simulink model "uart_xy_wiggler"  (R2018a)
settings: Solver=FixedStepDiscrete  StartTime=0.0  StopTime=inf  RelTol=1e-3
PreLoadFcn:
  | waijung.modelPreload; % Required for working with Waijung Blockset. Do not remove.
undefined symbols (not defined in the file or in its folder): HSEOSC, Link, LQFP144, ST, STM32F446ZE
libraries: simulink x10, commsynccomp2 x7, stm32f4_io_lib x3, dspstat3 x2, stm32f4_device_config_lib x1, dspbuff3 x1
(part 5 of 9)

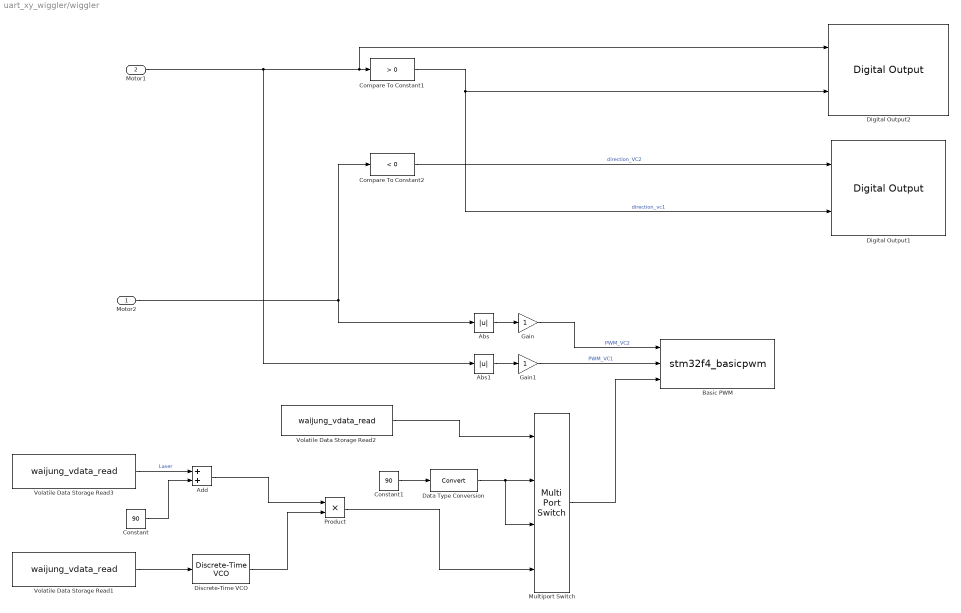
== system uart_xy_wiggler/wiggler ==
  Motor2 : Inport
  Motor1 : Inport  Port=2
  Abs : Abs
  Abs1 : Abs
  Add : Sum
  Basic PWM : S-Function  FunctionName=stm32f4_basicpwm  Parameters=timer,pwmperiod,ch1pin,ch2pin,ch3pin,ch4pin,sampletime,sampletimestr,blockid,apb,portstr,pinstr,pinmat,timarr,timprescale,chmat,polaritystr  SFunctionDeploymentMode=off  EnableBusSupport=off  mask(stm32f4_basicpwm){timer=3, pwmperiod=5.0000e-05, polarity=Active High, polaritystr=TIM_OCPolarity_High, ch1pin=Not available - Do not use, ch2pin=C7, ch3pin=C8, ch4pin=C9, sampletime=0.001, sampletimestr=-1, blockid=wigglerBasicPWM, portpinstr=,C7,C8,C9, enablecustomportlabel=off, cinputportlabel=In1, In2, In3, In4, coutputportlabel=0, apb=1, portstr=["C"], pinstr=["GPIO_Pin_7 | GPIO_Pin_8 | GPIO_Pin_9"], pinmat=[3 7 8 9], timarr=4499, timprescale=0, chmat=[2  3  4]}
      mask prompts: pwmperiod "PWM Period (seconds)"; ch1pin "Channel 1"; ch2pin "Channel 2"; ch3pin "Channel 3"; ch4pin "Channel 4"; sampletime "Sample time (sec)"; sampletimestr "Compiled sample time (sec) in string"; portpinstr "Port pin string"; enablecustomportlabel "Enable custom port labels"; cinputportlabel "Custom input port labels (Ex. In1, In2, In3)"; coutputportlabel "Custom output port labels (Ex. Out1, Out2, Out3)"; portstr "Port string"; pinstr "Pin string"; pinmat "Pin matrix"; timarr "Timer ARR"; timprescale "Timer PRESCALE"; chmat "Channel order"
      mask help:
      | This block implements basic Edge-aligned Pulse Width Modulation (PWM) generation.
      | All timers are 16-bit. The PWM period is fixed (per timer).
      mask init:
      | stm32f4_basicpwm_callback('init');
      mask Help: web(fullfile(waijungdocroot,'stm32f4_basicpwm.htm'),'-browser')
      mask TypeOptions timer: 1 | 2 | 3 | 4 | 5 | 8 | 9 | 10 | 11 | 12 | 13 | 14
      mask Callback timer: stm32f4_basicpwm_callback('timer');
      mask Callback pwmperiod: stm32f4_basicpwm_callback('pwmperiod');
      mask TypeOptions polarity: Active High | Active Low
      mask Callback polarity: stm32f4_basicpwm_callback('polarity');
      mask TypeOptions ch1pin: Not available - Do not use | A6 | B4 | C6
      mask Callback ch1pin: stm32f4_basicpwm_callback('ch1pin');
      mask TypeOptions ch2pin: Not available - Do not use | A7 | B5 | C7
      mask Callback ch2pin: stm32f4_basicpwm_callback('ch2pin');
      mask TypeOptions ch3pin: Not available - Do not use | B0 | C8
      mask Callback ch3pin: stm32f4_basicpwm_callback('ch3pin');
      mask TypeOptions ch4pin: Not available - Do not use | B1 | C9
      mask Callback ch4pin: stm32f4_basicpwm_callback('ch4pin');
      mask Callback sampletime: stm32f4_basicpwm_callback('sampletime');
      mask Callback sampletimestr: stm32f4_basicpwm_callback('sampletimestr');
      mask Callback blockid: stm32f4_basicpwm_callback('blockid');
      mask Callback enablecustomportlabel: stm32f4_basicpwm_callback('enablecustomportlabel');
      mask Display: text(0.95, 0.5, 'Timer: 3\nPolarity: Active High\nPeriod (sec) 5.0000e-05 \nTs (sec): -1','ver','middle','hor','right');port_label('input', 1,'CH2 (C7)');port_label('input', 2,'CH3 (C8)');port_label('input', 3,'CH4 (C9)')
  Compare To Constant1 : simulink/Logic and Bit Operations/Compare To Constant  relop=>  const=0  OutDataTypeStr=boolean
  Compare To Constant2 : simulink/Logic and Bit Operations/Compare To Constant  relop=<  const=0  OutDataTypeStr=boolean
  Constant : Constant  Value=90
  Constant1 : Constant  Value=90  SampleTime=0.01
  Data Type Conversion : DataTypeConversion
  Digital Output1 : stm32f4_io_lib/Digital Output  use_bitband=on  port=F  speed=100  porttype=Push Pull  porttypestr=PP  use_pin0=off  use_pin1=off  use_pin2=off  use_pin3=off  use_pin4=off  use_pin5=off  use_pin6=off  use_pin7=off  use_pin8=off  use_pin9=off  use_pin10=off  use_pin11=off  use_pin12=off  use_pin13=on  use_pin14=on  use_pin15=off  pinstr=GPIO_Pin_13 | GPIO_Pin_14  usedpinarray="[0  0  0  0  0  0  0  0  0  0  0  0  0  1  1  0]"  bitbandingstr=|  sampletime=-1  sampletimestr=-1  blockid=wigglerDigitalOutput1  enablecustomportlabel=off  globalinit=off  cinputportlabel=In1, In2  coutputportlabel=0
      | #define wigglerDigitalOutput1_F13 Peripheral_BB(GPIOF->ODR, 13)  /* Output pin */
      | #define wigglerDigitalOutput1_F14 Peripheral_BB(GPIOF->ODR, 14)  /* Output pin */
      settings: SourceProductName=Waijung Blockset
  Digital Output2 : stm32f4_io_lib/Digital Output  use_bitband=on  port=D  speed=100  porttype=Push Pull  porttypestr=PP  use_pin0=on  use_pin1=off  use_pin2=off  use_pin3=off  use_pin4=off  use_pin5=off  use_pin6=off  use_pin7=on  use_pin8=off  use_pin9=off  use_pin10=off  use_pin11=off  use_pin12=off  use_pin13=off  use_pin14=off  use_pin15=off  pinstr=GPIO_Pin_0 | GPIO_Pin_7  usedpinarray="[1  0  0  0  0  0  0  1  0  0  0  0  0  0  0  0]"  bitbandingstr=|  sampletime=-1  sampletimestr=-1  blockid=wigglerDigitalOutput2  enablecustomportlabel=off  globalinit=off  cinputportlabel=In1, In2  coutputportlabel=0
      | #define wigglerDigitalOutput2_D0 Peripheral_BB(GPIOD->ODR, 0)  /* Output pin */
      | #define wigglerDigitalOutput2_D7 Peripheral_BB(GPIOD->ODR, 7)  /* Output pin */
      settings: SourceProductName=Waijung Blockset
  Discrete-Time VCO : commsynccomp2/Discrete-Time VCO  Ac=1  Fc=0  Kc=1  Ph=0  ts=0.01
      settings: SourceProductName=Communications System Toolbox  SourceProductBaseCode=CM
  Gain : Gain
  Gain1 : Gain
  Multiport Switch : MultiPortSwitch  DataPortOrder=Zero-based contiguous  zeroidx=on
  Product : Product
  Volatile Data Storage Read1 : S-Function  FunctionName=waijung_vdata_read  Parameters=storagename,varname,sampletime,sampletimestr,blockid,storagetype,storagetypestr  SFunctionDeploymentMode=off  EnableBusSupport=off  mask(waijung_vdata_read){storagename=LissaFreq, varname=LissajousDataVolatileDataStorage8_LissaFreq, sampletime=.01, sampletimestr=-1, blockid=wigglerVolatileDataStorageRead1, storagetype=double, storagetypestr=double}
      mask prompts: storagename "Storage Name"; varname "Variable name"; sampletime "Sample time (sec)"; sampletimestr "Compiled sample time (sec) in string"; storagetype "Data type"; storagetypestr "Data type string"
      mask help: This block implements read data from a buffer.
      mask init:
      | waijung_vdata_read_callback('init');
      mask Help: web(fullfile(waijungdocroot,'Volatile_Data_Storage_Read.htm'))
      mask TypeOptions storagename: ab3 | ab1 | ab2 | ab4 | ab5 | ab6 | ab7 | ab8 | ab9 | ab10 | Ays | Ayc | Axs | A_Laser | LissaFreq | Axc | Laser | vcx | flag | CircleFlag | CircleFrequency | vcy | CircleR
      mask Callback storagename: waijung_vdata_read_callback('storagename');
      mask Callback varname: waijung_vdata_read_callback('varname');
      mask Callback sampletime: waijung_vdata_read_callback('sampletime');
      mask Callback sampletimestr: waijung_vdata_read_callback('sampletimestr');
      mask Callback blockid: waijung_vdata_read_callback('blockid');
      mask Callback storagetype: waijung_vdata_read_callback('storagetype');
      mask Display: text(0.05, 0.5, 'Buffer: LissaFreq','ver','middle','hor','left');port_label('output',1,'D1(double)')
  Volatile Data Storage Read2 : S-Function  FunctionName=waijung_vdata_read  Parameters=storagename,varname,sampletime,sampletimestr,blockid,storagetype,storagetypestr  SFunctionDeploymentMode=off  EnableBusSupport=off  mask(waijung_vdata_read){storagename=CircleFlag, varname=VolatileDataStorage4_CircleFlag, sampletime=.01, sampletimestr=-1, blockid=VolatileDataStorageRead2, storagetype=double, storagetypestr=double}
      mask prompts: storagename "Storage Name"; varname "Variable name"; sampletime "Sample time (sec)"; sampletimestr "Compiled sample time (sec) in string"; storagetype "Data type"; storagetypestr "Data type string"
      mask help: This block implements read data from a buffer.
      mask init:
      | waijung_vdata_read_callback('init');
      mask Help: web(fullfile(waijungdocroot,'Volatile_Data_Storage_Read.htm'))
      mask TypeOptions storagename: ab3 | ab1 | ab2 | ab4 | ab5 | ab6 | ab7 | ab8 | ab9 | ab10 | Ays | Ayc | Axs | A_Laser | LissaFreq | Axc | Laser | vcx | flag | CircleFlag | CircleFrequency | vcy | CircleR
      mask Callback storagename: waijung_vdata_read_callback('storagename');
      mask Callback varname: waijung_vdata_read_callback('varname');
      mask Callback sampletime: waijung_vdata_read_callback('sampletime');
      mask Callback sampletimestr: waijung_vdata_read_callback('sampletimestr');
      mask Callback blockid: waijung_vdata_read_callback('blockid');
      mask Callback storagetype: waijung_vdata_read_callback('storagetype');
      mask Display: text(0.05, 0.5, 'Buffer: CircleFlag','ver','middle','hor','left');port_label('output',1,'D1(double)')
  Volatile Data Storage Read3 : S-Function  FunctionName=waijung_vdata_read  Parameters=storagename,varname,sampletime,sampletimestr,blockid,storagetype,storagetypestr  SFunctionDeploymentMode=off  EnableBusSupport=off  mask(waijung_vdata_read){storagename=A_Laser, varname=LissajousDataVolatileDataStorage7_A_Laser, sampletime=.01, sampletimestr=-1, blockid=wigglerVolatileDataStorageRead3, storagetype=double, storagetypestr=double}
      mask prompts: storagename "Storage Name"; varname "Variable name"; sampletime "Sample time (sec)"; sampletimestr "Compiled sample time (sec) in string"; storagetype "Data type"; storagetypestr "Data type string"
      mask help: This block implements read data from a buffer.
      mask init:
      | waijung_vdata_read_callback('init');
      mask Help: web(fullfile(waijungdocroot,'Volatile_Data_Storage_Read.htm'))
      mask TypeOptions storagename: ab3 | ab1 | ab2 | ab4 | ab5 | ab6 | ab7 | ab8 | ab9 | ab10 | Ays | Ayc | Axs | A_Laser | LissaFreq | Axc | Laser | vcx | flag | CircleFlag | CircleFrequency | vcy | CircleR
      mask Callback storagename: waijung_vdata_read_callback('storagename');
      mask Callback varname: waijung_vdata_read_callback('varname');
      mask Callback sampletime: waijung_vdata_read_callback('sampletime');
      mask Callback sampletimestr: waijung_vdata_read_callback('sampletimestr');
      mask Callback blockid: waijung_vdata_read_callback('blockid');
      mask Callback storagetype: waijung_vdata_read_callback('storagetype');
      mask Display: text(0.05, 0.5, 'Buffer: A_Laser','ver','middle','hor','left');port_label('output',1,'D1(double)')
  wires:
  Gain1/1 -> Basic PWM/2  "PWM_VC1"
  Gain/1 -> Basic PWM/1  "PWM_VC2"
  Compare To Constant1/1 -> Digital Output1/2, Digital Output2/2  "direction_vc1"
  Compare To Constant2/1 -> Digital Output1/1  "direction_VC2"
  Abs/1 -> Gain/1
  Abs1/1 -> Gain1/1
  Motor2/1 -> Compare To Constant2/1, Abs/1
  Motor1/1 -> Digital Output2/1, Compare To Constant1/1, Abs1/1
  Volatile Data Storage Read3/1 -> Add/1  "Laser"
  Constant/1 -> Add/2
  Volatile Data Storage Read1/1 -> Discrete-Time VCO/1
  Add/1 -> Product/1
  Discrete-Time VCO/1 -> Product/2
  Volatile Data Storage Read2/1 -> Multiport Switch/1
  Product/1 -> Multiport Switch/4
  Constant1/1 -> Data Type Conversion/1
  Multiport Switch/1 -> Basic PWM/3
  Data Type Conversion/1 -> Multiport Switch/3, Multiport Switch/2

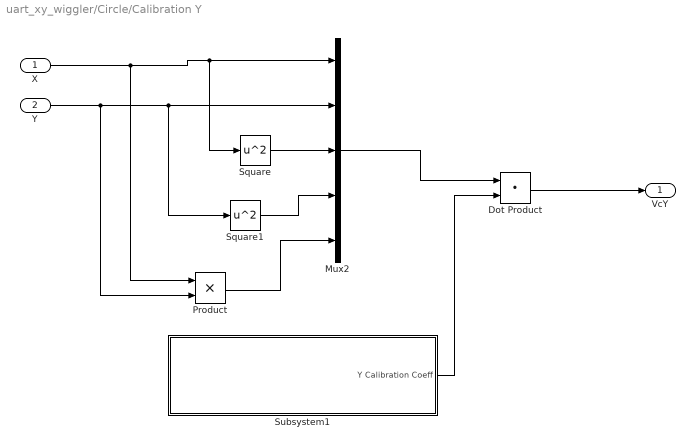
== system uart_xy_wiggler/Circle/Calibration Y ==
  X : Inport
  Y : Inport  Port=2
  Dot Product : DotProduct  InputSameDT=on  OutDataTypeStr=Inherit: Inherit via internal rule
  Mux2 : Mux  Inputs=5
  Product : Product
  Square : Math  Operator=square  SaturateOnIntegerOverflow=on
  Square1 : Math  Operator=square  SaturateOnIntegerOverflow=on
  Subsystem1 : Subsystem
  VcY : Outport
  wires:
  X/1 -> Product/1, Square/1, Mux2/1
  Y/1 -> Product/2, Square1/1, Mux2/2
  Square/1 -> Mux2/3
  Square1/1 -> Mux2/4
  Product/1 -> Mux2/5
  Mux2/1 -> Dot Product/1
  Dot Product/1 -> VcY/1
  Subsystem1/1(Y Calibration Coeff) -> Dot Product/2

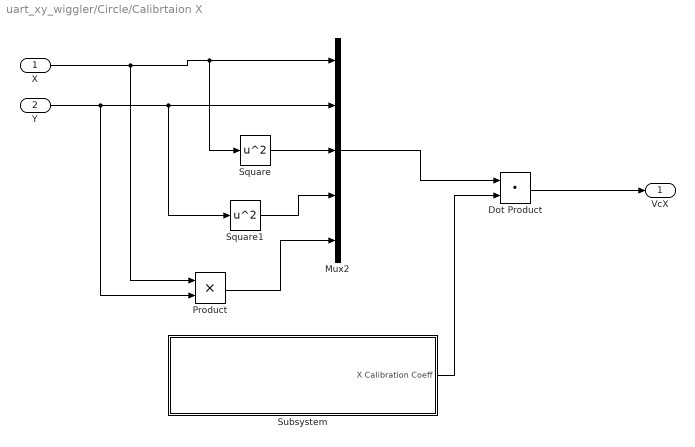
== system uart_xy_wiggler/Circle/Calibrtaion X ==
  X : Inport
  Y : Inport  Port=2
  Dot Product : DotProduct  InputSameDT=on  OutDataTypeStr=Inherit: Inherit via internal rule
  Mux2 : Mux  Inputs=5
  Product : Product
  Square : Math  Operator=square  SaturateOnIntegerOverflow=on
  Square1 : Math  Operator=square  SaturateOnIntegerOverflow=on
  Subsystem : Subsystem
  VcX : Outport
  wires:
  X/1 -> Product/1, Square/1, Mux2/1
  Y/1 -> Product/2, Square1/1, Mux2/2
  Square/1 -> Mux2/3
  Square1/1 -> Mux2/4
  Product/1 -> Mux2/5
  Mux2/1 -> Dot Product/1
  Dot Product/1 -> VcX/1
  Subsystem/1(X Calibration Coeff) -> Dot Product/2

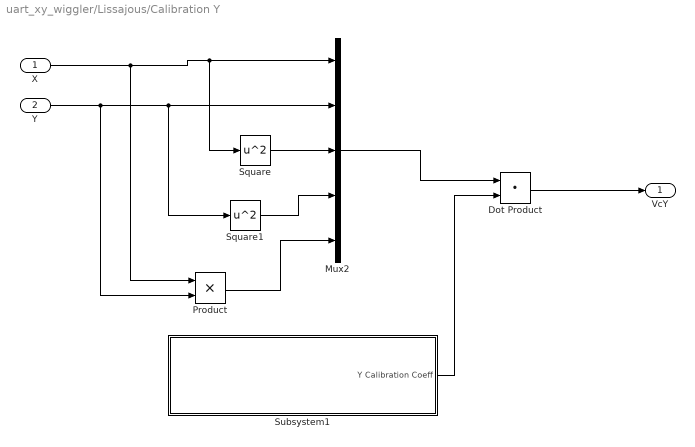
== system uart_xy_wiggler/Lissajous/Calibration Y ==
  X : Inport
  Y : Inport  Port=2
  Dot Product : DotProduct  InputSameDT=on  OutDataTypeStr=Inherit: Inherit via internal rule
  Mux2 : Mux  Inputs=5
  Product : Product
  Square : Math  Operator=square  SaturateOnIntegerOverflow=on
  Square1 : Math  Operator=square  SaturateOnIntegerOverflow=on
  Subsystem1 : Subsystem
  VcY : Outport
  wires:
  X/1 -> Product/1, Square/1, Mux2/1
  Y/1 -> Product/2, Square1/1, Mux2/2
  Square/1 -> Mux2/3
  Square1/1 -> Mux2/4
  Product/1 -> Mux2/5
  Mux2/1 -> Dot Product/1
  Dot Product/1 -> VcY/1
  Subsystem1/1(Y Calibration Coeff) -> Dot Product/2

== system uart_xy_wiggler/Lissajous/Calibrtaion X ==
  X : Inport
  Y : Inport  Port=2
  Dot Product : DotProduct  InputSameDT=on  OutDataTypeStr=Inherit: Inherit via internal rule
  Mux2 : Mux  Inputs=5
  Product : Product
  Square : Math  Operator=square  SaturateOnIntegerOverflow=on
  Square1 : Math  Operator=square  SaturateOnIntegerOverflow=on
  Subsystem : Subsystem
  VcX : Outport
  wires:
  X/1 -> Product/1, Square/1, Mux2/1
  Y/1 -> Product/2, Square1/1, Mux2/2
  Square/1 -> Mux2/3
  Square1/1 -> Mux2/4
  Product/1 -> Mux2/5
  Mux2/1 -> Dot Product/1
  Dot Product/1 -> VcX/1
  Subsystem/1(X Calibration Coeff) -> Dot Product/2

== system uart_xy_wiggler/record_and_send_via_UART/Subsystem3 ==
  In1 : Inport
  Enable : EnablePort
  Demux : Demux
  UART Tx3 : S-Function  Priority=1  FunctionName=stm32f4_usart  Parameters=configuration,uartmodule,transfer,baudrate,inputtype,outputtype,confstr,binheaderarray,binterminatorarray,asciiheader,asciiterminator,bindatalength,packetmode,varname,sampletime,sampletimestr,blockid  SFunctionDeploymentMode=off  EnableBusSupport=off  mask(stm32f4_usart){configuration=Tx, uartmodule=3, baudrate=115200, databits=8, parity=No, stopbit=1, remaptxpin=Not used, remaprxpin=Not used, flowcontrol=None, remapctspin=Not used, remaprtspin=Not used, advanceoptions=off, rxbuffersize=512, txbuffersize=512, transfer=Non-Blocking, packetmode=Binary, binheader='7E 7E', binterminator='03 03', porttype_double=0, porttype_single=4, porttype_int8=0, porttype_uint8=0, porttype_int16=0, porttype_uint16=0, porttype_int32=0, porttype_uint32=0, asciiformat='flag = %u Num=%u empty=%d full=%d', rx_asciiterminator=CRLF (0x0D 0x0A - "\r\n"), tx_asciiterminator=CRLF (0x0D 0x0A - "\r\n"), storagename=<empty>, varname=, inputtype=[4  1 1 1 1], outputtype=[0], binheaderarray=[2 126  126], binterminatorarray=[2 3  3], bindatalength=16, asciiheader='flag = %u Num=%u empty=%d full=%d\r\n', asciiterminator=[2 13 10], sampletime=1e-3, sampletimestr=-1, blockid=record_and_send_via_UARTSubsystem3UARTTx3, confstr=[ "dummy", "0", "*", "*", "0", "*", "*", "0", "*", "*", "0", "*", "*", "1", "4", "3", "1", "4", "1", "512", "512", "1", "3", "115200", "8", "No", "1", "None", "USART3"], lastmodule=1}
      mask prompts: uartmodule "UART Module"; baudrate "Baud rate (bps)"; databits "Data bits"; stopbit "Stop bit"; remaptxpin "Tx Pin"; remaprxpin "Rx Pin"; flowcontrol "Hardware flow control"; remapctspin "HW Flow control, CTS Pin"; remaprtspin "HW Flow control, RTS Pin"; advanceoptions "Advance options"; rxbuffersize "Rx buffer size (bytes)"; txbuffersize "Tx buffer size (bytes)"; packetmode "Packet mode"; binheader "Binary header (example: '7E 7E')"; binterminator "Binary terminator (example: '03 03')"; porttype_double "Number of data port, type DOUBLE"; porttype_single "Number of data port, type SINGLE"; porttype_int8 "Number of data port, type INT8"; porttype_uint8 "Number of data port, type UINT8"; porttype_int16 "Number of data port, type INT16"; porttype_uint16 "Number of data port, type UINT16"; porttype_int32 "Number of data port, type INT32"; porttype_uint32 "Number of data port, type UINT32"; asciiformat "Ascii format"; rx_asciiterminator "End of packet"; tx_asciiterminator "End of packet"; storagename "Buffer"; varname "Var name"; inputtype "Input data type"; outputtype "Output data type"; binheaderarray "Binary header"; binterminatorarray "Binary terminator"; bindatalength "Binary data length"; asciiheader "Ascii header (printf format)"; asciiterminator "Ascii terminator"; sampletime "Sample time (sec)"; sampletimestr "Compiled sample time (sec) in string"; confstr "Configuration string"; lastmodule "Last module selected"
      mask help:
      | Data type for Ascii format
      | %u, %i, %d, %o, %x: uint32
      | %e, %g, %f: single
      | %c: int8
      mask init:
      | stm32f4_usart_callback('init');
      mask Help: web(fullfile(waijungdocroot,'stm32f4_usart_tx.htm'), '-browser')
      mask TypeOptions configuration: Setup | Tx | Rx
      mask Callback configuration: stm32f4_usart_callback('configuration');
      mask TypeOptions uartmodule: 1 | 2 | 3 | 4 | 5 | 6
      mask Callback uartmodule: stm32f4_usart_callback('uartmodule');
      mask Callback baudrate: stm32f4_usart_callback('baudrate');
      mask TypeOptions databits: 8
      mask TypeOptions parity: No | Odd | Even
      mask TypeOptions stopbit: 0.5 | 1 | 1.5 | 2
      mask TypeOptions remaptxpin: Not used | A9 | B6
      mask TypeOptions remaprxpin: Not used | A10 | B7
      mask TypeOptions flowcontrol: None | RTS | CTS | RTS/CTS
      mask Callback flowcontrol: stm32f4_usart_callback('flowcontrol');
      mask TypeOptions remapctspin: Not used | A11
      mask TypeOptions remaprtspin: Not used | A12
      mask Callback advanceoptions: stm32f4_usart_callback('advanceoptions');
      mask TypeOptions rxbuffersize: 16 | 32 | 64 | 128 | 256 | 512 | 1024 | 2048
      mask TypeOptions txbuffersize: 16 | 32 | 64 | 128 | 256 | 512 | 1024 | 2048
      mask TypeOptions transfer: Blocking | Non-Blocking
      mask Callback transfer: stm32f4_usart_callback('transfer');
      mask TypeOptions packetmode: Ascii | Binary | Binary Vector | String Buffer | Raw Buffer
      mask Callback packetmode: stm32f4_usart_callback('packetmode');
      mask Callback binheader: stm32f4_usart_callback('binheader');
      mask Callback binterminator: stm32f4_usart_callback('binterminator');
      mask Callback porttype_double: stm32f4_usart_callback('porttype');
      mask Callback porttype_single: stm32f4_usart_callback('porttype');
      mask Callback porttype_int8: stm32f4_usart_callback('porttype');
      mask Callback porttype_uint8: stm32f4_usart_callback('porttype');
      mask Callback porttype_int16: stm32f4_usart_callback('porttype');
      mask Callback porttype_uint16: stm32f4_usart_callback('porttype');
      mask Callback porttype_int32: stm32f4_usart_callback('porttype');
      mask Callback porttype_uint32: stm32f4_usart_callback('porttype');
      mask Callback asciiformat: stm32f4_usart_callback('asciiformat');
      mask TypeOptions rx_asciiterminator: CR (0x0D - "\r") | LF (0x0A - "\n") | CRLF (0x0D 0x0A - "\r\n")
      mask Callback rx_asciiterminator: stm32f4_usart_callback('rx_asciiterminator');
      mask TypeOptions tx_asciiterminator: CR (0x0D - "\r") | LF (0x0A - "\n") | CRLF (0x0D 0x0A - "\r\n") | None
      mask Callback tx_asciiterminator: stm32f4_usart_callback('tx_asciiterminator');
      mask TypeOptions storagename: <empty>
      mask Callback storagename: stm32f4_usart_callback('storagename');
      mask Callback varname: stm32f4_usart_callback('varname');
      mask Callback sampletime: stm32f4_usart_callback('sampletime');
      mask Callback sampletimestr: stm32f4_usart_callback('sampletimestr');
      mask Callback blockid: stm32f4_usart_callback('blockid');
      mask Display: text(0.5, 0.5, 'Module: USART3_Tx\nPacket: Binary\nTransfer: Non-Blocking\nTs (sec): -1','ver','middle','hor','center'); port_label('input', 1,'single'); port_label('input', 2,'single'); port_label('input', 3,'single'); port_label('input', 4,'single');
  wires:
  In1/1 -> Demux/1
  Demux/1 -> UART Tx3/1
  Demux/2 -> UART Tx3/2
  Demux/3 -> UART Tx3/3
  Demux/4 -> UART Tx3/4

== system uart_xy_wiggler/record_and_send_via_UART/set flag=0 ==
  Enable : EnablePort
  Constant : Constant  Value=0  OutDataTypeStr=uint8
  Volatile Data Storage Write : S-Function  FunctionName=waijung_vdata_write  Parameters=storagename,varname,sampletime,sampletimestr,blockid,storagetype,storagetypestr  SFunctionDeploymentMode=off  EnableBusSupport=off  mask(waijung_vdata_write){storagename=flag, varname=VolatileDataStorage3_flag, sampletime=0.1, sampletimestr=-1, blockid=record_and_send_via_UARTsetflag0VolatileDataStorageWrite, storagetype=uint8, storagetypestr=uint8_t}
      mask prompts: storagename "Storage Name"; varname "Variable name"; sampletime "Sample time (sec)"; sampletimestr "Compiled sample time (sec) in string"; storagetype "Data type"; storagetypestr "Data type string"
      mask help: This block implements write data to a buffer.
      mask init:
      | waijung_vdata_write_callback('init');
      mask Help: web(fullfile(waijungdocroot,'Volatile_Data_Storage_Write.htm'))
      mask TypeOptions storagename: ab3 | ab1 | ab2 | ab4 | ab5 | ab6 | ab7 | ab8 | ab9 | ab10 | Ays | Ayc | Axs | A_Laser | LissaFreq | Axc | Laser | vcx | flag | CircleFlag | CircleFrequency | vcy | CircleR
      mask Callback storagename: waijung_vdata_write_callback('storagename');
      mask Callback varname: waijung_vdata_write_callback('varname');
      mask Callback sampletime: waijung_vdata_write_callback('sampletime');
      mask Callback sampletimestr: waijung_vdata_write_callback('sampletimestr');
      mask Callback blockid: waijung_vdata_write_callback('blockid');
      mask Callback storagetype: waijung_vdata_write_callback('storagetype');
      mask Display: text(0.95, 0.5, 'Buffer: flag','ver','middle','hor','right');port_label('input',1,'D1(uint8)')
  wires:
  Constant/1 -> Volatile Data Storage Write/1
